simulink model "OptimalControl"  (R2018b)
settings: Solver=VariableStepAuto  StartTime=0.0  StopTime=6  RelTol=1e-3
values from neighbouring files (symbols this model uses):
  K = -lqr(sys_A, sys_B, Q, R)    [LQRadjuster.m]
  x0 = [20*pi/180;0;0;0]    [LQRadjuster.m]
undefined symbols (not defined in the file or in its folder): sys_A, sys_B
settings Model: Creator=kuwano  LastModifiedBy=ku_sk

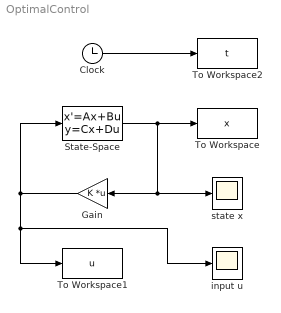
== system OptimalControl ==
  Clock : Clock
  Gain : Gain  Gain=K  Multiplication=Matrix(K*u)
  State-Space : StateSpace  A=sys_A  B=sys_B  C=eye(4)  D=zeros(4,1)  InitialCondition=x0
  To Workspace : ToWorkspace  VariableName=x  SampleTime=-1
  To Workspace1 : ToWorkspace  VariableName=u  SampleTime=-1
  To Workspace2 : ToWorkspace  VariableName=t  SaveFormat=Timeseries  SampleTime=-1
  input u : Scope
  state x : Scope
  wires:
  State-Space/1 -> To Workspace/1, Gain/1, state x/1
  Clock/1 -> To Workspace2/1
  Gain/1 -> State-Space/1, input u/1, To Workspace1/1
